simulink model "slGTC_3gdl"  (Simulink 9.1)
settings: Solver=ode45  StartTime=0.0  StopTime=2  MaxStep=1e-3  RelTol=1e-8  EnableMultiTasking=on
undefined symbols (not defined in the file or in its folder): CinematicaDirecta
settings Model: Creator=Manuel G. Ortega  LastModifiedBy=usuario  ExtModeTrigMode=oneshot  ExtModeArmWhenConnect=off
settings DataIOCC: SignalLoggingSaveFormat=ModelDataLogs
settings OptimizationCC: BooleanDataType=off  ExpressionDepthLimit=2147483647  InitFltsAndDblsToZero=on
settings DebuggingCC: SaveWithParameterizedLinksMsg=none  SignalResolutionControl=TryResolveAllWithWarning  MultiTaskDSMMsg=warning  MultiTaskCondExecSysMsg=none  FcnCallInpInsideContextMsg=warning  StateNameClashWarn=warning
settings HardwareCC: TargetUnknown=on
settings GRTTargetCC: TargetFcnLib=ansi_tfl_tmw.mat  GeneratePreprocessorConditionals=Disable all
settings ConfigComp: CovSFcnEnable=off

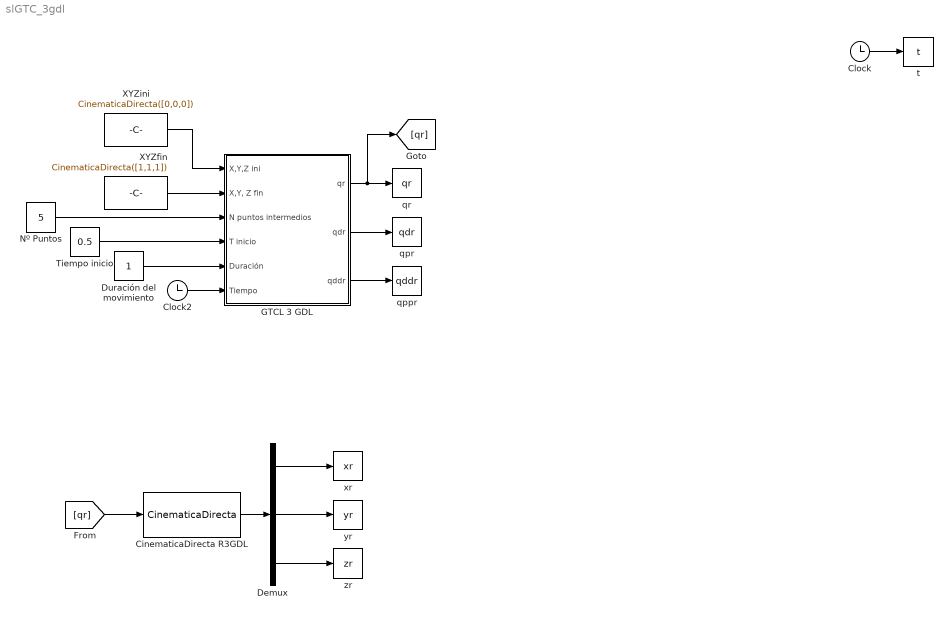
== system slGTC_3gdl ==
  CinematicaDirecta R3GDL : MATLABFcn  MATLABFcn=CinematicaDirecta
  Clock : Clock
  Clock2 : Clock
  Demux : Demux  Outputs=3
  Duración del movimiento : Constant
  GTCL 3 GDL : Subsystem
  Nº Puntos : Constant  Value=5
  Tiempo inicio : Constant  Value=0.5
  XYZfin : Constant  Value=CinematicaDirecta([1,1,1])
  XYZini : Constant  Value=CinematicaDirecta([0,0,0])
  qppr : ToWorkspace  VariableName=qddr  SampleTime=-1
  qpr : ToWorkspace  VariableName=qdr  SampleTime=-1
  qr : ToWorkspace  VariableName=qr  SampleTime=-1
  t : ToWorkspace  VariableName=t  SampleTime=-1
  xr : ToWorkspace  VariableName=xr  SampleTime=-1
  yr : ToWorkspace  VariableName=yr  SampleTime=-1
  zr : ToWorkspace  VariableName=zr  SampleTime=-1
  wires:
  Clock/1 -> t/1
  Clock2/1 -> GTCL 3 GDL/6(Tiempo)
  Duración del movimiento/1 -> GTCL 3 GDL/5(Duración)
  Tiempo inicio/1 -> GTCL 3 GDL/4(T inicio)
  Nº Puntos/1 -> GTCL 3 GDL/3(N puntos intermedios)
  XYZfin/1 -> GTCL 3 GDL/2("X,Y, Z fin")
  XYZini/1 -> GTCL 3 GDL/1(X,Y,Z ini)
  GTCL 3 GDL/1(qr) -> qr/1, [qr]
  GTCL 3 GDL/2(qdr) -> qpr/1
  GTCL 3 GDL/3(qddr) -> qppr/1
  [qr] -> CinematicaDirecta R3GDL/1
  CinematicaDirecta R3GDL/1 -> Demux/1
  Demux/1 -> xr/1
  Demux/2 -> yr/1
  Demux/3 -> zr/1

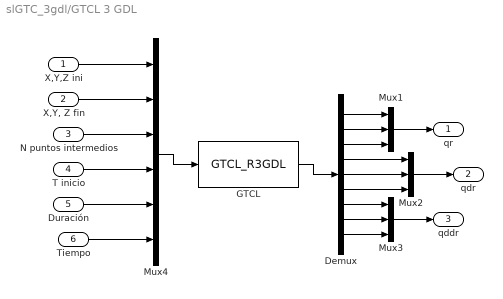
== system slGTC_3gdl/GTCL 3 GDL ==
  X,Y,Z ini : Inport
  "X,Y, Z fin" : Inport  Port=2
  N puntos intermedios : Inport  Port=3
  T inicio : Inport  Port=4
  Duración : Inport  Port=5
  Tiempo : Inport  Port=6
  Demux : Demux  Outputs=9
  GTCL : MATLABFcn  MATLABFcn=GTCL_R3GDL  OutputDimensions=9
  Mux1 : Mux  Inputs=3
  Mux2 : Mux  Inputs=3
  Mux3 : Mux  Inputs=3
  Mux4 : Mux  Inputs=6
  qr : Outport
  qdr : Outport  Port=2
  qddr : Outport  Port=3
  wires:
  Mux1/1 -> qr/1
  Mux4/1 -> GTCL/1
  X,Y,Z ini/1 -> Mux4/1
  "X,Y, Z fin"/1 -> Mux4/2
  N puntos intermedios/1 -> Mux4/3
  T inicio/1 -> Mux4/4
  Duración/1 -> Mux4/5
  Tiempo/1 -> Mux4/6
  GTCL/1 -> Demux/1
  Demux/1 -> Mux1/1
  Demux/2 -> Mux1/2
  Demux/3 -> Mux1/3
  Mux2/1 -> qdr/1
  Demux/4 -> Mux2/1
  Demux/5 -> Mux2/2
  Demux/6 -> Mux2/3
  Mux3/1 -> qddr/1
  Demux/7 -> Mux3/1
  Demux/8 -> Mux3/2
  Demux/9 -> Mux3/3
